simulink model "transmitancja"  (R2023a)
settings: Solver=VariableStepAuto  StartTime=0.0  StopTime=10.0  RelTol=1e-3
settings Model: Creator=adams  LastModifiedBy=adams

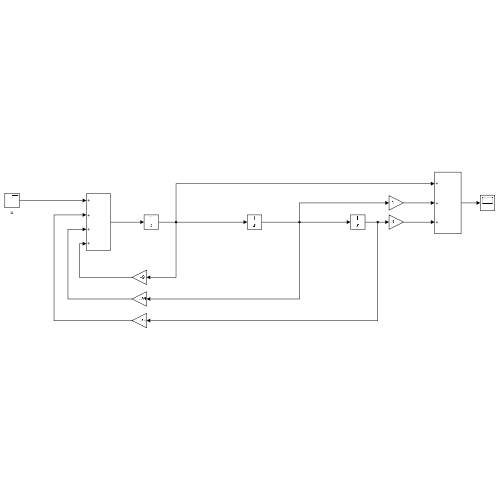
[thumbnail: Simulink's stored preview of the top-level diagram]
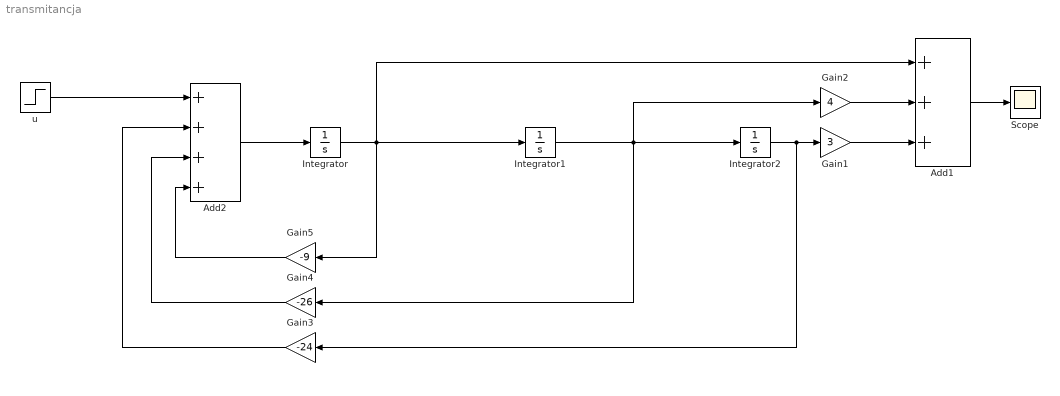
== system transmitancja ==
  Add1 : Sum  Inputs=+++
  Add2 : Sum  Inputs=++++
  Gain1 : Gain  Gain=3
  Gain2 : Gain  Gain=4
  Gain3 : Gain  Gain=-24
  Gain4 : Gain  Gain=-26
  Gain5 : Gain  Gain=-9
  Integrator : Integrator
  Integrator1 : Integrator
  Integrator2 : Integrator
  Scope : Scope
  u : Step  SampleTime=0
  wires:
  Integrator/1 -> Add1/1, Integrator1/1, Gain5/1
  Integrator1/1 -> Gain4/1, Gain2/1, Integrator2/1
  Gain1/1 -> Add1/3
  Integrator2/1 -> Gain3/1, Gain1/1
  Gain2/1 -> Add1/2
  u/1 -> Add2/1
  Add2/1 -> Integrator/1
  Gain5/1 -> Add2/4
  Gain4/1 -> Add2/3
  Gain3/1 -> Add2/2
  Add1/1 -> Scope/1
